simulink library "SUB_ECU_L4_MABX_HW_Interface_PIC_PB"  (R2018a)
settings: Solver=VariableStepAuto  StartTime=0.0  StopTime=10.0  RelTol=1e-3
PostLoadFcn:
  | , if any(exist('dsrtsu_mdlpostloadfcn', 'file') == [2, 3, 6]), try dsrtsu_mdlpostloadfcn('Execute', bdroot); catch fprintf('Error in PostLoadFcn (dsrtsu_mdlpostloadfcn) for model "%s":\n %s\n', bdroot, lasterr); end, end,
undefined symbols (not defined in the file or in its folder): CANR_PROPB_REAX_3_13_CHANNEL_APV, CANR_PROPB_REAX_4_13_CHANNEL_APV, CANR_PROPB_XPR_1_50_CHANNEL_APV, ENUM_CAN_RX_T, ENUM_CAN_TX_T, ENUM_REAX_OPERATION_MODE_T, ENUM_SIGNAL_HEALTH_T, ENUM_XBR_CONTROL_MODE_T, ENUM_XBR_EBI_MODE_T, ENUM_XBR_PASS_THROUGH_ACTIVE_T, ENUM_XBR_PRIORITY_T, ENUM_XPR_INHIBIT_PARK_MANUAL_T, ENUM_XPR_INHIBIT_UNPARK_MANUAL_T, ENUM_XPR_PARK_MANUAL_T, ENUM_XPR_UNPARK_MANUAL_T, PROPB_REAX_1_E4_DES_POS_SIG_SRC_APV, PROPB_REAX_1_E4_DESIRED_OPMODE_APV, PROPB_REAX_1_E4_DESIRED_POSITION_APV, PROPB_REAX_CHANNEL_APV, ptc_matlab_lib
libraries: PTC_MBDS_LIB x293, rtican x158, simulink x61, EmE_MBD_Blockset x38, rti1401lib_dio_type4 x14, simulink_need_slupdate x7, $bdroot x5, rti1401lib_adc_type4 x3, rtmapslib x3, dsa_tcpip_lib x2, SUB_ECU_L4_MABX_HW_Interface_PTC_1571 x1, rtitasklib x1
(part 32 of 49)

== system SUB_ECU_L4_MABX_HW_Interface_PIC_PB/INPUTS_PIC_PB/CAN_PIC_PB/CAN_RX_EBC1_0B/RX_CAN_1_EBC1 ==
  Enable : Inport
  Bus Creator3 : BusCreator  Inputs=25
  Data Type Conversion10 : DataTypeConversion  OutDataTypeStr=double  SaturateOnIntegerOverflow=on
  Data Type Conversion8 : DataTypeConversion  OutDataTypeStr=boolean  SaturateOnIntegerOverflow=on
  Data Type Conversion9 : DataTypeConversion  OutDataTypeStr=double  SaturateOnIntegerOverflow=on
  EBC1_0B : rtican/RTICAN Receive (RX)   Reserved1=[]  Reserved2=[]  Reserved3=[]  Reserved4=[]  SfcnMessage=[]  Msg_Struct=[]  BoardTypeNo=[]  BoardNo=[]  ChannelNo=[]  Parameters=[]  DialogFcn=[]  UnitName=[]  Revision=[]  UnitValues=[]  DSProperties=struct('RTI',struct('Version',uint32(5),'BlockType',struct('isSLSource',uint8(1),'isSLSink',uint8(1),'isHWSource',uint8(0),'isHWSink',uint8(0),'isSetup',uint8(0),'isInline',uint8(1),'isNonInline',uint8(0),'isInterrupt',uint8(0),'isChannelwise',uint8(0)),'IOBoardType','RTICAN','UnitType','MESSAGE','Identifier','RX','DialogType','MSVC','BlockSet','RTICAN','SlaveProcessor','CAN'))  RTIBlockInterface=struct('OutputPortsWidth',int32([1 1 1 1 1 1 1 1 1 1 1 1 1 1 1 1 1 1 1 1 1 1 1 1 1]),'OutputPortsActive',ones(1,25),'OutputPortsName',{{'ASREngCtrlActive','ASRBrakeCtrlActive','AntiLockBrakingActive','EBSBrakeSwitch','BrakePedalPos','ABSOffroadSwitch','ASROffroadSwitch','ASRHillHolderSwitch','TractionCtrlOverrideSwitch','AccelInterlockSwitch','EngDerateSwitch','EngAuxShutdownSwitch','RemoteAccelEnableSwitch','EngRetarderSelection','ABSFullyOperational','EBSRedWarningSignal','ABS_EBSAmberWarningSignal','ATC_ASRInformationSignal','SrcAddrssOfCtrllngDvcFrBrkCntrl','HaltBrakeSwitch','TrailerABSStatus','TrctrMntdTrilerABSWarningSignal',['RX status'],['RX time'],['RX delta time']}},'OutputPortsDataType',{{'SS_DOUBLE','SS_DOUBLE','SS_DOUBLE','SS_DOUBLE','SS_DOUBLE','SS_DOUBLE','SS_DOUBLE','SS_DOUBLE','SS_DOUBLE','SS_DOUBLE','SS_DOUBLE','SS_DOUBLE','SS_DOUBLE','SS_DOUBLE','SS_DOUBLE','SS_DOUBLE','SS_DOUBLE','SS_DOUBLE','SS_DOUBLE','SS_DOUBLE','SS_DOUBLE','SS_DOUBLE','SS_DOUBLE','SS_DOUBLE','SS_DOUBLE'}},'OutputPortsLabel',{{'ASREngCtrlActive','ASRBrakeCtrlActive','AntiLockBrakingActive','EBSBrakeSwitch','BrakePedalPos','ABSOffroadSwitch','ASROffroadSwitch','ASRHillHolderSwitch','TractionCtrlOverrideSwitch','AccelInterlockSwitch','EngDerateSwitch','EngAuxShutdownSwitch','RemoteAccelEnableSwitch','EngRetarderSelection','ABSFullyOperational','EBSRedWarningSignal','ABS_EBSAmberWarningSignal','ATC_ASRInformationSignal','SrcAddrssOfCtrllngDvcFrBrkCntrl','HaltBrakeSwitch','TrailerABSStatus','TrctrMntdTrilerABSWarningSignal','','',''}},'OutputPortsLabelMode','ON','InputPortsWidth',int32(0),'InputPortsActive',0,'DialogFcn','rtican_message_interface_gui','BlockDisplay',{{'','center'}},'IconTransparency','on','ParameterTunableNames',{{}},'InitLevel',3,'BlockName',struct('Token',{{'EBC1_0B'}}),'SampleTime',{{-1}},'TriggerPort',{{'none'}},'EnablePort',{{'yes'}})  RTIBlockParameters=struct('BoardTypeNo',{{1,'OFF',[]}},'BoardNo',{{1,'ON',[1 16]}},'ChannelNo',{{1,'ON',[1 2]}},'Parameters',{{struct('DataFileSupport',struct('DataFileSelectedMaster',1,'DataFileSelectedLocal',0,'DataFileName','c:\localdata\chris\advanced_tech\adas\level4_rcp\truck1571\dbc\mabx_can1.dbc|','DataFileDate',{{{['02-May-2017 14:24:53']},{['10-Feb-2017 15:17:28']}}},'SelectedFile',['<no file selected>']),'Options',struct('StatusSelected',1,'TimeSelected',1,'DeltaTimeSelected',1,'BytePortSelected',0,'MessageLengthSelected',0,'TriggerPort',struct('Selected',0,'TriggerType',0),'UserCoding',struct('Selected',0,'InterfaceFile','UserDecodingFile','FcnName','UserDecodeFcn','InportSelected',0,'InportWidth',1,'OutportSelected',0,'OutportWidth',1),'EnablePortSelected',1,'SignalOnPortnameSelected',1,'UseRXService',1),'Message',struct('MsgOnBlocknameSelected',1,'MsgName','EBC1_0B','MsgIdFormat',1,'MsgId',418382091,'MsgLength',8,'NumSignals',22,'SampleTime',-1,'Signal',struct('SgnName',{'ASREngCtrlActive','ASRBrakeCtrlActive','AntiLockBrakingActive','EBSBrakeSwitch','BrakePedalPos','ABSOffroadSwitch','ASROffroadSwitch','ASRHillHolderSwitch','TractionCtrlOverrideSwitch','AccelInterlockSwitch','EngDerateSwitch','EngAuxShutdownSwitch','RemoteAccelEnableSwitch','EngRetarderSelection','ABSFullyOperational','EBSRedWarningSignal','ABS_EBSAmberWarningSignal','ATC_ASRInformationSignal','SrcAddrssOfCtrllngDvcFrBrkCntrl','HaltBrakeSwitch','TrailerABSStatus','TrctrMntdTrilerABSWarningSignal'},'SgnStartBit',{0,2,4,6,8,16,18,20,22,24,26,28,30,32,40,42,44,46,48,58,60,62},'SgnLength',{2,2,2,2,8,2,2,2,2,2,2,2,2,8,2,2,2,2,8,2,2,2},'SgnType',{0,0,0,0,0,0,0,0,0,0,0,0,0,0,0,0,0,0,0,0,0,0},'ModeValue',{-1,-1,-1,-1,-1,-1,-1,-1,-1,-1,-1,-1,-1,-1,-1,-1,-1,-1,-1,-1,-1,-1},'DataType',{0,0,0,0,0,0,0,0,0,0,0,0,0,0,0,0,0,0,0,0,0,0},'ByteLayout',{0,0,0,0,0,0,0,0,0,0,0,0,0,0,0,0,0,0,0,0,0,0},'Factor',{1,1,1,1,0.4,1,1,1,1,1,1,1,1,0.4,1,1,1,1,1,1,1,1},'Offset',{0,0,0,0,0,0,0,0,0,0,0,0,0,0,0,0,0,0,0,0,0,0},'SgnComment',{{['State signal which indicates that ASR engine control has been commanded to be active.']},{['State signal which indicates that ASR brake control is active.']},{['State signal which indicates that the ABS is active.']},{['Switch signal which indicates that the brake pedal is being pressed.']},{['Ratio of brake pedal position to maximum pedal position.']},{['Switch signal which indicates the position of the ABS off-road switch.']},{['Switch signal which indicates the position of the ASR off-road switch.']},{['Switch signal which indicates the position of the ASR “hill holder” switch.']},{['Switch signal which indicates the position of the traction control override switch.']},{['Switch signal used to disable the accelerator and remote accelerator inputs, causing the engine to return to idle.']},{['Switch signal used to activate the torque limiting feature of the engine.']},{['Switch signal which requests that all engine fueling stop.']},{['Switch signal which indicates that the remote accelerator has been enabled and controls the engine.']},{['The position of the operator controlled selector, expressed as a percentage and determined by the ratio of the current']},{['Signal which indicates whether an ABS system is fully operational or whether its functionality is reduced by a defect or by']},{['This parameter commands the EBS red optical warning signal']},{['This parameter commands the ABS/EBS amber/yellow optical warning signal']},{['This parameter commands the ATC/ASR driver information signal, for example a dash lamp.']},{['The source address of the SAE J1939 device currently controlling the brake system.']},{['Switch signal which indicates the position of the halt brake switch.']},{['State signal which indicates that ABS in the trailer is actively controlling the brakes.']},{['This parameter commands the tractor-mounted trailer ABS optical warning signal.']}},'SgnUnit',{'','','','','%','','','','','','','','','%','','','','','','','',''},'Min',{0,0,0,0,0,0,0,0,0,0,0,0,0,0,0,0,0,0,0,0,0,0},'Max',{3,3,3,3,100,3,3,3,3,3,3,3,3,100,3,3,3,3,255,3,3,3},'SLDataType',{'SS_DOUBLE','SS_DOUBLE','SS_DOUBLE','SS_DOUBLE','SS_DOUBLE','SS_DOUBLE','SS_DOUBLE','SS_DOUBLE','SS_DOUBLE','SS_DOUBLE','SS_DOUBLE','SS_DOUBLE','SS_DOUBLE','SS_DOUBLE','SS_DOUBLE','SS_DOUBLE','SS_DOUBLE','SS_DOUBLE','SS_DOUBLE','SS_DOUBLE','SS_DOUBLE','SS_DOUBLE'}),'MsgIdNumFormat',1,'MsgComment',{{['Electronic Brake Controller 1']}}),'Version',1.2,'general',struct('isFromLib',0)),'OFF',[]}},'GroupId',{{struct('Group',{{'RTICAN'}},'No',1,'Behavior',{{'NAMECHANGE'}},'BlockType',{{'SINK'}},'NameChangeFlag',0),'OFF',[]}},'SFcnRTICANMessage',{{struct('MsgType','RX','SFcnPortType','Scalar','MsgName','EBC1_0B','MsgIdFormat','XTD','MsgId',418382091,'MsgLength',8,'NumSignals',22,'SampleTime',-1,'Signal',struct('SgnName',{'ASREngCtrlActive','ASRBrakeCtrlActive','AntiLockBrakingActive','EBSBrakeSwitch','BrakePedalPos','ABSOffroadSwitch','ASROffroadSwitch','ASRHillHolderSwitch','TractionCtrlOverrideSwitch','AccelInterlockSwitch','EngDerateSwitch','EngAuxShutdownSwitch','RemoteAccelEnableSwitch','EngRetarderSelection','ABSFullyOperational','EBSRedWarningSignal','ABS_EBSAmberWarningSignal','ATC_ASRInformationSignal','SrcAddrssOfCtrllngDvcFrBrkCntrl','HaltBrakeSwitch','TrailerABSStatus','TrctrMntdTrilerABSWarningSignal'},'SgnStartBit',{0,2,4,6,8,16,18,20,22,24,26,28,30,32,40,42,44,46,48,58,60,62},'SgnLength',{2,2,2,2,8,2,2,2,2,2,2,2,2,8,2,2,2,2,8,2,2,2},'SgnType',{'standard','standard','standard','standard','standard','standard','standard','standard','standard','standard','standard','standard','standard','standard','standard','standard','standard','standard','standard','standard','standard','standard'},'ModeValue',{-1,-1,-1,-1,-1,-1,-1,-1,-1,-1,-1,-1,-1,-1,-1,-1,-1,-1,-1,-1,-1,-1},'DataType',{['unsigned int'],['unsigned int'],['unsigned int'],['unsigned int'],['unsigned int'],['unsigned int'],['unsigned int'],['unsigned int'],['unsigned int'],['unsigned int'],['unsigned int'],['unsigned int'],['unsigned int'],['unsigned int'],['unsigned int'],['unsigned int'],['unsigned int'],['unsigned int'],['unsigned int'],['unsigned int'],['unsigned int'],['unsigned int']},'ByteLayout',{['little endian'],['little endian'],['little endian'],['little endian'],['little endian'],['little endian'],['little endian'],['little endian'],['little endian'],['little endian'],['little endian'],['little endian'],['little endian'],['little endian'],['little endian'],['little endian'],['little endian'],['little endian'],['little endian'],['little endian'],['little endian'],['little endian']},'Factor',{1,1,1,1,0.4,1,1,1,1,1,1,1,1,0.4,1,1,1,1,1,1,1,1},'Offset',{0,0,0,0,0,0,0,0,0,0,0,0,0,0,0,0,0,0,0,0,0,0},'SLDataType',{'SS_DOUBLE','SS_DOUBLE','SS_DOUBLE','SS_DOUBLE','SS_DOUBLE','SS_DOUBLE','SS_DOUBLE','SS_DOUBLE','SS_DOUBLE','SS_DOUBLE','SS_DOUBLE','SS_DOUBLE','SS_DOUBLE','SS_DOUBLE','SS_DOUBLE','SS_DOUBLE','SS_DOUBLE','SS_DOUBLE','SS_DOUBLE','SS_DOUBLE','SS_DOUBLE','SS_DOUBLE'}),'StatusSelected','yes','TimeSelected','yes','DeltaTimeSelected','yes','BytePortSelected','no','MessageLengthSelected','no','TriggerPort',struct('Selected','no','TriggerType',0),'UserCoding',struct('Selected','no','InterfaceFile','UserDecodingFile','FcnName','UserDecodeFcn','InportSelected','no','InportWidth',1,'OutportSelected','no','OutportWidth',1),'EnablePortSelected','yes','UseRXService','yes','BoardType','DS1','BoardNo',3,'ControllerNo',1),'OFF',[]}},'TLCFileName',{{'rtican_rx_message','OFF',[]}})  RTISFcnParameters=struct('SFcnRTICANMessage','struct','TLCFileName','char')  RTIBlockParaDefault=struct('BoardTypeNo',4302,'BoardNo',1,'ChannelNo',1,'Parameters',struct('DataFileSupport',struct('DataFileSelectedMaster',0,'DataFileSelectedLocal',0,'DataFileName','','DataFileDate','','SelectedFile',['<no file selected>']),'Options',struct('StatusSelected',1,'TimeSelected',1,'DeltaTimeSelected',1,'BytePortSelected',0,'MessageLengthSelected',0,'TriggerPort',struct('Selected',0,'TriggerType','rising'),'UserCoding',struct('Selected',0,'InterfaceFile','UserDecodingFile','FcnName','UserDecodeFcn','InportSelected',0,'InportWidth',1,'OutportSelected',0,'OutportWidth',1),'EnablePortSelected',0,'SignalOnPortnameSelected',1,'UseRXService',0),'Message',struct('MsgOnBlocknameSelected',0,'MsgName',['RX Message'],'MsgIdFormat',0,'MsgId',100,'MsgLength',8,'NumSignals',1,'SampleTime',-1,'Signal',struct('SgnName',['RX signal'],'SgnStartBit',0,'SgnLength',8,'SgnType',0,'ModeValue',-1,'DataType',0,'SLDataType','SS_DOUBLE','ByteLayout',0,'Factor',1,'Offset',0,'Min',0,'Max',255,'SgnComment',{{}},'SgnUnit',''),'MsgIdNumFormat',0,'MsgComment',{{''}}),'Version',1.2,'general',struct('isFromLib',1)),'GroupId',struct('Group',{{'RTICAN'}},'No',1,'Behavior',{{'NAMECHANGE'}},'BlockType',{{'SINK'}},'NameChangeFlag',0),'SFcnRTICANMessage',struct('MsgType','RX','MsgName',['RX Message'],'MsgIdFormat','STD','MsgId',100,'MsgLength',8,'NumSignals',1,'SampleTime',-1,'Signal',struct('SgnName',['RX signal'],'SgnStartBit',0,'SgnLength',8,'SgnType','standard','ModeValue',-1,'DataType',['unsigned int'],'ByteLayout',['little endian'],'SLDataType','SS_DOUBLE','Factor',1,'Offset',0),'StatusSelected','yes','TimeSelected','yes','DeltaTimeSelected','yes','BytePortSelected','no','MessageLengthSelected','no','EnablePortSelected','no','UserCoding',struct('Selected','no','InterfaceFile','UserDecodingFile','FcnName','UserDecodeFcn','InportSelected','no','InportWidth',1,'OutportSelected','no','OutportWidth',1),'TriggerPort',struct('Selected','no','TriggerType','rising'),'UseRXService','no','BoardType','DS4302','BoardNo',1,'ControllerNo',1,'SFcnPortType','Scalar'),'TLCFileName','rtican_rx_message')
      settings: AttributesFormatString=Group Id: RTICAN1\n  SourceProductName=dSPACE RTI CAN Blockset
  EBC1_0B_ : Outport
  wires:
  EBC1_0B/7 -> Bus Creator3/7  "ASROffroadSwitch"
  EBC1_0B/6 -> Bus Creator3/6  "ABSOffroadSwitch"
  EBC1_0B/5 -> Bus Creator3/5  "BrakePedalPos"
  EBC1_0B/4 -> Bus Creator3/4  "EBSBrakeSwitch"
  EBC1_0B/3 -> Bus Creator3/3  "AntiLockBrakingActive"
  EBC1_0B/2 -> Bus Creator3/2  "ASRBrakeCtrlActive"
  EBC1_0B/1 -> Bus Creator3/1  "ASREngCtrlActive"
  EBC1_0B/9 -> Bus Creator3/9  "TractionCtrlOverrideSwitch"
  EBC1_0B/22 -> Bus Creator3/22  "TrctrMntdTrilerABSWarningSignal"
  EBC1_0B/21 -> Bus Creator3/21  "TrailerABSStatus"
  EBC1_0B/20 -> Bus Creator3/20  "HaltBrakeSwitch"
  EBC1_0B/19 -> Bus Creator3/19  "SrcAddrssOfCtrllngDvcFrBrkCntrl"
  EBC1_0B/18 -> Bus Creator3/18  "ATC_ASRInformationSignal"
  EBC1_0B/17 -> Bus Creator3/17  "ABS_EBSAmberWarningSignal"
  EBC1_0B/16 -> Bus Creator3/16  "EBSRedWarningSignal"
  EBC1_0B/15 -> Bus Creator3/15  "ABSFullyOperational"
  EBC1_0B/14 -> Bus Creator3/14  "EngRetarderSelection"
  EBC1_0B/13 -> Bus Creator3/13  "RemoteAccelEnableSwitch"
  EBC1_0B/12 -> Bus Creator3/12  "EngAuxShutdownSwitch"
  EBC1_0B/11 -> Bus Creator3/11  "EngDerateSwitch"
  EBC1_0B/10 -> Bus Creator3/10  "AccelInterlockSwitch"
  EBC1_0B/8 -> Bus Creator3/8  "ASRHillHolderSwitch"
  Data Type Conversion9/1 -> Bus Creator3/24  "RX_time"
  Data Type Conversion10/1 -> Bus Creator3/25  "RX_delta_time"
  Data Type Conversion8/1 -> Bus Creator3/23  "RX_status"
  EBC1_0B/23 -> Data Type Conversion8/1
  EBC1_0B/24 -> Data Type Conversion9/1
  EBC1_0B/25 -> Data Type Conversion10/1
  Enable/1 -> EBC1_0B/Enable
  Bus Creator3/1 -> EBC1_0B_/1  "EBC1_0B"

== system SUB_ECU_L4_MABX_HW_Interface_PIC_PB/INPUTS_PIC_PB/CAN_PIC_PB/CAN_RX_EBC1_8B/RX_CAN_5_EBC1 ==
  Enable : Inport
  Bus Creator3 : BusCreator  Inputs=25
  Data Type Conversion10 : DataTypeConversion  OutDataTypeStr=double  SaturateOnIntegerOverflow=on
  Data Type Conversion8 : DataTypeConversion  OutDataTypeStr=boolean  SaturateOnIntegerOverflow=on
  Data Type Conversion9 : DataTypeConversion  OutDataTypeStr=double  SaturateOnIntegerOverflow=on
  EBC1_0B : rtican/RTICAN Receive (RX)   Reserved1=[]  Reserved2=[]  Reserved3=[]  Reserved4=[]  SfcnMessage=[]  Msg_Struct=[]  BoardTypeNo=[]  BoardNo=[]  ChannelNo=[]  Parameters=[]  DialogFcn=[]  UnitName=[]  Revision=[]  UnitValues=[]  DSProperties=struct('RTI',struct('Version',uint32(5),'BlockType',struct('isSLSource',uint8(1),'isSLSink',uint8(1),'isHWSource',uint8(0),'isHWSink',uint8(0),'isSetup',uint8(0),'isInline',uint8(1),'isNonInline',uint8(0),'isInterrupt',uint8(0),'isChannelwise',uint8(0)),'IOBoardType','RTICAN','UnitType','MESSAGE','Identifier','RX','DialogType','MSVC','BlockSet','RTICAN','SlaveProcessor','CAN'))  RTIBlockInterface=struct('OutputPortsWidth',int32([1 1 1 1 1 1 1 1 1 1 1 1 1 1 1 1 1 1 1 1 1 1 1 1 1]),'OutputPortsActive',ones(1,25),'OutputPortsName',{{'ASREngCtrlActive','ASRBrakeCtrlActive','AntiLockBrakingActive','EBSBrakeSwitch','BrakePedalPos','ABSOffroadSwitch','ASROffroadSwitch','ASRHillHolderSwitch','TractionCtrlOverrideSwitch','AccelInterlockSwitch','EngDerateSwitch','EngAuxShutdownSwitch','RemoteAccelEnableSwitch','EngRetarderSelection','ABSFullyOperational','EBSRedWarningSignal','ABS_EBSAmberWarningSignal','ATC_ASRInformationSignal','SrcAddrssOfCtrllngDvcFrBrkCntrl','HaltBrakeSwitch','TrailerABSStatus','TrctrMntdTrilerABSWarningSignal',['RX status'],['RX time'],['RX delta time']}},'OutputPortsDataType',{{'SS_DOUBLE','SS_DOUBLE','SS_DOUBLE','SS_DOUBLE','SS_DOUBLE','SS_DOUBLE','SS_DOUBLE','SS_DOUBLE','SS_DOUBLE','SS_DOUBLE','SS_DOUBLE','SS_DOUBLE','SS_DOUBLE','SS_DOUBLE','SS_DOUBLE','SS_DOUBLE','SS_DOUBLE','SS_DOUBLE','SS_DOUBLE','SS_DOUBLE','SS_DOUBLE','SS_DOUBLE','SS_DOUBLE','SS_DOUBLE','SS_DOUBLE'}},'OutputPortsLabel',{{'ASREngCtrlActive','ASRBrakeCtrlActive','AntiLockBrakingActive','EBSBrakeSwitch','BrakePedalPos','ABSOffroadSwitch','ASROffroadSwitch','ASRHillHolderSwitch','TractionCtrlOverrideSwitch','AccelInterlockSwitch','EngDerateSwitch','EngAuxShutdownSwitch','RemoteAccelEnableSwitch','EngRetarderSelection','ABSFullyOperational','EBSRedWarningSignal','ABS_EBSAmberWarningSignal','ATC_ASRInformationSignal','SrcAddrssOfCtrllngDvcFrBrkCntrl','HaltBrakeSwitch','TrailerABSStatus','TrctrMntdTrilerABSWarningSignal','','',''}},'OutputPortsLabelMode','ON','InputPortsWidth',int32(0),'InputPortsActive',0,'DialogFcn','rtican_message_interface_gui','BlockDisplay',{{'','center'}},'IconTransparency','on','ParameterTunableNames',{{}},'InitLevel',3,'BlockName',struct('Token',{{'EBC1_0B'}}),'SampleTime',{{-1}},'TriggerPort',{{'none'}},'EnablePort',{{'yes'}})  RTIBlockParameters=struct('BoardTypeNo',{{1,'OFF',[]}},'BoardNo',{{1,'ON',[1 16]}},'ChannelNo',{{2,'ON',[1 2]}},'Parameters',{{struct('DataFileSupport',struct('DataFileSelectedMaster',1,'DataFileSelectedLocal',0,'DataFileName',['c:\users\gavin.coelho\repos\l4 svn\branches\gennaro\project_l4\src\projectlibrary\dbc\mabx_can2.dbc|'],'DataFileDate',{{{['02-May-2017 14:24:53']},{['10-Feb-2017 15:17:28']}}},'SelectedFile',['<no file selected>']),'Options',struct('StatusSelected',1,'TimeSelected',1,'DeltaTimeSelected',1,'BytePortSelected',0,'MessageLengthSelected',0,'TriggerPort',struct('Selected',0,'TriggerType',0),'UserCoding',struct('Selected',0,'InterfaceFile','UserDecodingFile','FcnName','UserDecodeFcn','InportSelected',0,'InportWidth',1,'OutportSelected',0,'OutportWidth',1),'EnablePortSelected',1,'SignalOnPortnameSelected',1,'UseRXService',1),'Message',struct('MsgOnBlocknameSelected',1,'MsgName','EBC1_0B','MsgIdFormat',1,'MsgId',418382219,'MsgLength',8,'NumSignals',22,'SampleTime',-1,'Signal',struct('SgnName',{'ASREngCtrlActive','ASRBrakeCtrlActive','AntiLockBrakingActive','EBSBrakeSwitch','BrakePedalPos','ABSOffroadSwitch','ASROffroadSwitch','ASRHillHolderSwitch','TractionCtrlOverrideSwitch','AccelInterlockSwitch','EngDerateSwitch','EngAuxShutdownSwitch','RemoteAccelEnableSwitch','EngRetarderSelection','ABSFullyOperational','EBSRedWarningSignal','ABS_EBSAmberWarningSignal','ATC_ASRInformationSignal','SrcAddrssOfCtrllngDvcFrBrkCntrl','HaltBrakeSwitch','TrailerABSStatus','TrctrMntdTrilerABSWarningSignal'},'SgnStartBit',{0,2,4,6,8,16,18,20,22,24,26,28,30,32,40,42,44,46,48,58,60,62},'SgnLength',{2,2,2,2,8,2,2,2,2,2,2,2,2,8,2,2,2,2,8,2,2,2},'SgnType',{0,0,0,0,0,0,0,0,0,0,0,0,0,0,0,0,0,0,0,0,0,0},'ModeValue',{-1,-1,-1,-1,-1,-1,-1,-1,-1,-1,-1,-1,-1,-1,-1,-1,-1,-1,-1,-1,-1,-1},'DataType',{0,0,0,0,0,0,0,0,0,0,0,0,0,0,0,0,0,0,0,0,0,0},'ByteLayout',{0,0,0,0,0,0,0,0,0,0,0,0,0,0,0,0,0,0,0,0,0,0},'Factor',{1,1,1,1,0.4,1,1,1,1,1,1,1,1,0.4,1,1,1,1,1,1,1,1},'Offset',{0,0,0,0,0,0,0,0,0,0,0,0,0,0,0,0,0,0,0,0,0,0},'SgnComment',{{['State signal which indicates that ASR engine control has been commanded to be active.']},{['State signal which indicates that ASR brake control is active.']},{['State signal which indicates that the ABS is active.']},{['Switch signal which indicates that the brake pedal is being pressed.']},{['Ratio of brake pedal position to maximum pedal position.']},{['Switch signal which indicates the position of the ABS off-road switch.']},{['Switch signal which indicates the position of the ASR off-road switch.']},{['Switch signal which indicates the position of the ASR “hill holder” switch.']},{['Switch signal which indicates the position of the traction control override switch.']},{['Switch signal used to disable the accelerator and remote accelerator inputs, causing the engine to return to idle.']},{['Switch signal used to activate the torque limiting feature of the engine.']},{['Switch signal which requests that all engine fueling stop.']},{['Switch signal which indicates that the remote accelerator has been enabled and controls the engine.']},{['The position of the operator controlled selector, expressed as a percentage and determined by the ratio of the current']},{['Signal which indicates whether an ABS system is fully operational or whether its functionality is reduced by a defect or by']},{['This parameter commands the EBS red optical warning signal']},{['This parameter commands the ABS/EBS amber/yellow optical warning signal']},{['This parameter commands the ATC/ASR driver information signal, for example a dash lamp.']},{['The source address of the SAE J1939 device currently controlling the brake system.']},{['Switch signal which indicates the position of the halt brake switch.']},{['State signal which indicates that ABS in the trailer is actively controlling the brakes.']},{['This parameter commands the tractor-mounted trailer ABS optical warning signal.']}},'SgnUnit',{'','','','','%','','','','','','','','','%','','','','','','','',''},'Min',{0,0,0,0,0,0,0,0,0,0,0,0,0,0,0,0,0,0,0,0,0,0},'Max',{3,3,3,3,100,3,3,3,3,3,3,3,3,100,3,3,3,3,255,3,3,3},'SLDataType',{'SS_DOUBLE','SS_DOUBLE','SS_DOUBLE','SS_DOUBLE','SS_DOUBLE','SS_DOUBLE','SS_DOUBLE','SS_DOUBLE','SS_DOUBLE','SS_DOUBLE','SS_DOUBLE','SS_DOUBLE','SS_DOUBLE','SS_DOUBLE','SS_DOUBLE','SS_DOUBLE','SS_DOUBLE','SS_DOUBLE','SS_DOUBLE','SS_DOUBLE','SS_DOUBLE','SS_DOUBLE'}),'MsgIdNumFormat',1,'MsgComment',{{['Electronic Brake Controller 1']}}),'Version',1.2,'general',struct('isFromLib',0)),'OFF',[]}},'GroupId',{{struct('Group',{{'RTICAN'}},'No',2,'Behavior',{{'NAMECHANGE'}},'BlockType',{{'SINK'}},'NameChangeFlag',0),'OFF',[]}},'SFcnRTICANMessage',{{struct('MsgType','RX','SFcnPortType','Scalar','MsgName','EBC1_0B','MsgIdFormat','XTD','MsgId',418382219,'MsgLength',8,'NumSignals',22,'SampleTime',-1,'Signal',struct('SgnName',{'ASREngCtrlActive','ASRBrakeCtrlActive','AntiLockBrakingActive','EBSBrakeSwitch','BrakePedalPos','ABSOffroadSwitch','ASROffroadSwitch','ASRHillHolderSwitch','TractionCtrlOverrideSwitch','AccelInterlockSwitch','EngDerateSwitch','EngAuxShutdownSwitch','RemoteAccelEnableSwitch','EngRetarderSelection','ABSFullyOperational','EBSRedWarningSignal','ABS_EBSAmberWarningSignal','ATC_ASRInformationSignal','SrcAddrssOfCtrllngDvcFrBrkCntrl','HaltBrakeSwitch','TrailerABSStatus','TrctrMntdTrilerABSWarningSignal'},'SgnStartBit',{0,2,4,6,8,16,18,20,22,24,26,28,30,32,40,42,44,46,48,58,60,62},'SgnLength',{2,2,2,2,8,2,2,2,2,2,2,2,2,8,2,2,2,2,8,2,2,2},'SgnType',{'standard','standard','standard','standard','standard','standard','standard','standard','standard','standard','standard','standard','standard','standard','standard','standard','standard','standard','standard','standard','standard','standard'},'ModeValue',{-1,-1,-1,-1,-1,-1,-1,-1,-1,-1,-1,-1,-1,-1,-1,-1,-1,-1,-1,-1,-1,-1},'DataType',{['unsigned int'],['unsigned int'],['unsigned int'],['unsigned int'],['unsigned int'],['unsigned int'],['unsigned int'],['unsigned int'],['unsigned int'],['unsigned int'],['unsigned int'],['unsigned int'],['unsigned int'],['unsigned int'],['unsigned int'],['unsigned int'],['unsigned int'],['unsigned int'],['unsigned int'],['unsigned int'],['unsigned int'],['unsigned int']},'ByteLayout',{['little endian'],['little endian'],['little endian'],['little endian'],['little endian'],['little endian'],['little endian'],['little endian'],['little endian'],['little endian'],['little endian'],['little endian'],['little endian'],['little endian'],['little endian'],['little endian'],['little endian'],['little endian'],['little endian'],['little endian'],['little endian'],['little endian']},'Factor',{1,1,1,1,0.4,1,1,1,1,1,1,1,1,0.4,1,1,1,1,1,1,1,1},'Offset',{0,0,0,0,0,0,0,0,0,0,0,0,0,0,0,0,0,0,0,0,0,0},'SLDataType',{'SS_DOUBLE','SS_DOUBLE','SS_DOUBLE','SS_DOUBLE','SS_DOUBLE','SS_DOUBLE','SS_DOUBLE','SS_DOUBLE','SS_DOUBLE','SS_DOUBLE','SS_DOUBLE','SS_DOUBLE','SS_DOUBLE','SS_DOUBLE','SS_DOUBLE','SS_DOUBLE','SS_DOUBLE','SS_DOUBLE','SS_DOUBLE','SS_DOUBLE','SS_DOUBLE','SS_DOUBLE'}),'StatusSelected','yes','TimeSelected','yes','DeltaTimeSelected','yes','BytePortSelected','no','MessageLengthSelected','no','TriggerPort',struct('Selected','no','TriggerType',0),'UserCoding',struct('Selected','no','InterfaceFile','UserDecodingFile','FcnName','UserDecodeFcn','InportSelected','no','InportWidth',1,'OutportSelected','no','OutportWidth',1),'EnablePortSelected','yes','UseRXService','yes','BoardType','DS1','BoardNo',3,'ControllerNo',1),'OFF',[]}},'TLCFileName',{{'rtican_rx_message','OFF',[]}})  RTISFcnParameters=struct('SFcnRTICANMessage','struct','TLCFileName','char')  RTIBlockParaDefault=struct('BoardTypeNo',4302,'BoardNo',1,'ChannelNo',1,'Parameters',struct('DataFileSupport',struct('DataFileSelectedMaster',0,'DataFileSelectedLocal',0,'DataFileName','','DataFileDate','','SelectedFile',['<no file selected>']),'Options',struct('StatusSelected',1,'TimeSelected',1,'DeltaTimeSelected',1,'BytePortSelected',0,'MessageLengthSelected',0,'TriggerPort',struct('Selected',0,'TriggerType','rising'),'UserCoding',struct('Selected',0,'InterfaceFile','UserDecodingFile','FcnName','UserDecodeFcn','InportSelected',0,'InportWidth',1,'OutportSelected',0,'OutportWidth',1),'EnablePortSelected',0,'SignalOnPortnameSelected',1,'UseRXService',0),'Message',struct('MsgOnBlocknameSelected',0,'MsgName',['RX Message'],'MsgIdFormat',0,'MsgId',100,'MsgLength',8,'NumSignals',1,'SampleTime',-1,'Signal',struct('SgnName',['RX signal'],'SgnStartBit',0,'SgnLength',8,'SgnType',0,'ModeValue',-1,'DataType',0,'SLDataType','SS_DOUBLE','ByteLayout',0,'Factor',1,'Offset',0,'Min',0,'Max',255,'SgnComment',{{}},'SgnUnit',''),'MsgIdNumFormat',0,'MsgComment',{{''}}),'Version',1.2,'general',struct('isFromLib',1)),'GroupId',struct('Group',{{'RTICAN'}},'No',1,'Behavior',{{'NAMECHANGE'}},'BlockType',{{'SINK'}},'NameChangeFlag',0),'SFcnRTICANMessage',struct('MsgType','RX','MsgName',['RX Message'],'MsgIdFormat','STD','MsgId',100,'MsgLength',8,'NumSignals',1,'SampleTime',-1,'Signal',struct('SgnName',['RX signal'],'SgnStartBit',0,'SgnLength',8,'SgnType','standard','ModeValue',-1,'DataType',['unsigned int'],'ByteLayout',['little endian'],'SLDataType','SS_DOUBLE','Factor',1,'Offset',0),'StatusSelected','yes','TimeSelected','yes','DeltaTimeSelected','yes','BytePortSelected','no','MessageLengthSelected','no','EnablePortSelected','no','UserCoding',struct('Selected','no','InterfaceFile','UserDecodingFile','FcnName','UserDecodeFcn','InportSelected','no','InportWidth',1,'OutportSelected','no','OutportWidth',1),'TriggerPort',struct('Selected','no','TriggerType','rising'),'UseRXService','no','BoardType','DS4302','BoardNo',1,'ControllerNo',1,'SFcnPortType','Scalar'),'TLCFileName','rtican_rx_message')
      settings: AttributesFormatString=Group Id: RTICAN2\n  SourceProductName=dSPACE RTI CAN Blockset
  EBC1_8B : Outport
  wires:
  Bus Creator3/1 -> EBC1_8B/1  "EBC1_8B"
  Enable/1 -> EBC1_0B/Enable
  EBC1_0B/25 -> Data Type Conversion10/1
  EBC1_0B/24 -> Data Type Conversion9/1
  EBC1_0B/23 -> Data Type Conversion8/1
  Data Type Conversion8/1 -> Bus Creator3/23  "RX_status"
  Data Type Conversion10/1 -> Bus Creator3/25  "RX_delta_time"
  Data Type Conversion9/1 -> Bus Creator3/24  "RX_time"
  EBC1_0B/8 -> Bus Creator3/8  "ASRHillHolderSwitch"
  EBC1_0B/10 -> Bus Creator3/10  "AccelInterlockSwitch"
  EBC1_0B/11 -> Bus Creator3/11  "EngDerateSwitch"
  EBC1_0B/12 -> Bus Creator3/12  "EngAuxShutdownSwitch"
  EBC1_0B/13 -> Bus Creator3/13  "RemoteAccelEnableSwitch"
  EBC1_0B/14 -> Bus Creator3/14  "EngRetarderSelection"
  EBC1_0B/15 -> Bus Creator3/15  "ABSFullyOperational"
  EBC1_0B/16 -> Bus Creator3/16  "EBSRedWarningSignal"
  EBC1_0B/17 -> Bus Creator3/17  "ABS_EBSAmberWarningSignal"
  EBC1_0B/18 -> Bus Creator3/18  "ATC_ASRInformationSignal"
  EBC1_0B/19 -> Bus Creator3/19  "SrcAddrssOfCtrllngDvcFrBrkCntrl"
  EBC1_0B/20 -> Bus Creator3/20  "HaltBrakeSwitch"
  EBC1_0B/21 -> Bus Creator3/21  "TrailerABSStatus"
  EBC1_0B/22 -> Bus Creator3/22  "TrctrMntdTrilerABSWarningSignal"
  EBC1_0B/9 -> Bus Creator3/9  "TractionCtrlOverrideSwitch"
  EBC1_0B/1 -> Bus Creator3/1  "ASREngCtrlActive"
  EBC1_0B/2 -> Bus Creator3/2  "ASRBrakeCtrlActive"
  EBC1_0B/3 -> Bus Creator3/3  "AntiLockBrakingActive"
  EBC1_0B/4 -> Bus Creator3/4  "EBSBrakeSwitch"
  EBC1_0B/5 -> Bus Creator3/5  "BrakePedalPos"
  EBC1_0B/6 -> Bus Creator3/6  "ABSOffroadSwitch"
  EBC1_0B/7 -> Bus Creator3/7  "ASROffroadSwitch"

== system SUB_ECU_L4_MABX_HW_Interface_PIC_PB/INPUTS_PIC_PB/CAN_PIC_PB/CAN_RX_EBC2_0B/RX_CAN_1 ==
  Enable : Inport
  Bus Creator3 : BusCreator  Inputs=10
  Data Type Conversion10 : DataTypeConversion  OutDataTypeStr=double  SaturateOnIntegerOverflow=on
  Data Type Conversion8 : DataTypeConversion  OutDataTypeStr=boolean  SaturateOnIntegerOverflow=on
  Data Type Conversion9 : DataTypeConversion  OutDataTypeStr=double  SaturateOnIntegerOverflow=on
  EBC2_0B1 : rtican/RTICAN Receive (RX)   Reserved1=[]  Reserved2=[]  Reserved3=[]  Reserved4=[]  SfcnMessage=[]  Msg_Struct=[]  BoardTypeNo=[]  BoardNo=[]  ChannelNo=[]  Parameters=[]  DialogFcn=[]  UnitName=[]  Revision=[]  UnitValues=[]  DSProperties=struct('RTI',struct('Version',uint32(5),'BlockType',struct('isSLSource',uint8(1),'isSLSink',uint8(1),'isHWSource',uint8(0),'isHWSink',uint8(0),'isSetup',uint8(0),'isInline',uint8(1),'isNonInline',uint8(0),'isInterrupt',uint8(0),'isChannelwise',uint8(0)),'IOBoardType','RTICAN','UnitType','MESSAGE','Identifier','RX','DialogType','MSVC','BlockSet','RTICAN','SlaveProcessor','CAN'))  RTIBlockInterface=struct('OutputPortsWidth',int32([1 1 1 1 1 1 1 1 1 1]),'OutputPortsActive',[1 1 1 1 1 1 1 1 1 1],'OutputPortsName',{{'FrontAxleSpeed','RelativeSpeedFrontAxleLeftWheel','RlativeSpeedFrontAxleRightWheel','RelativeSpeedRearAxle1LeftWheel','RlativeSpeedRearAxle1RightWheel','RelativeSpeedRearAxle2LeftWheel','RlativeSpeedRearAxle2RightWheel',['RX status'],['RX time'],['RX delta time']}},'OutputPortsDataType',{{'SS_DOUBLE','SS_DOUBLE','SS_DOUBLE','SS_DOUBLE','SS_DOUBLE','SS_DOUBLE','SS_DOUBLE','SS_DOUBLE','SS_DOUBLE','SS_DOUBLE'}},'OutputPortsLabel',{{'FrontAxleSpeed','RelativeSpeedFrontAxleLeftWheel','RlativeSpeedFrontAxleRightWheel','RelativeSpeedRearAxle1LeftWheel','RlativeSpeedRearAxle1RightWheel','RelativeSpeedRearAxle2LeftWheel','RlativeSpeedRearAxle2RightWheel','','',''}},'OutputPortsLabelMode','ON','InputPortsWidth',int32(0),'InputPortsActive',0,'DialogFcn','rtican_message_interface_gui','BlockDisplay',{{'','center'}},'IconTransparency','on','ParameterTunableNames',{{}},'InitLevel',3,'BlockName',struct('Token',{{'EBC2_0B'}}),'SampleTime',{{-1}},'TriggerPort',{{'none'}},'EnablePort',{{'yes'}})  RTIBlockParameters=struct('BoardTypeNo',{{1,'OFF',[]}},'BoardNo',{{1,'ON',[1 16]}},'ChannelNo',{{1,'ON',[1 2]}},'Parameters',{{struct('DataFileSupport',struct('DataFileSelectedMaster',1,'DataFileSelectedLocal',1,'DataFileName','c:\localdata\chris\advanced_tech\adas\level4_rcp\truck1571\dbc\j1939_famosdbcwithfusion.dbc|','DataFileDate',{{{['03-Apr-2017 12:55:40']}}},'SelectedFile','dbc\j1939_famosdbcwithfusion.dbc'),'Options',struct('StatusSelected',1,'TimeSelected',1,'DeltaTimeSelected',1,'BytePortSelected',0,'MessageLengthSelected',0,'TriggerPort',struct('Selected',0,'TriggerType',0),'UserCoding',struct('Selected',0,'InterfaceFile','UserDecodingFile','FcnName','UserDecodeFcn','InportSelected',0,'InportWidth',1,'OutportSelected',0,'OutportWidth',1),'EnablePortSelected',1,'SignalOnPortnameSelected',1,'UseRXService',1),'Message',struct('MsgOnBlocknameSelected',1,'MsgName','EBC2_0B','MsgIdFormat',1,'MsgId',419348235,'MsgLength',8,'NumSignals',7,'SampleTime',-1,'Signal',struct('SgnName',{'FrontAxleSpeed','RelativeSpeedFrontAxleLeftWheel','RlativeSpeedFrontAxleRightWheel','RelativeSpeedRearAxle1LeftWheel','RlativeSpeedRearAxle1RightWheel','RelativeSpeedRearAxle2LeftWheel','RlativeSpeedRearAxle2RightWheel'},'SgnStartBit',{0,16,24,32,40,48,56},'SgnLength',{16,8,8,8,8,8,8},'SgnType',{0,0,0,0,0,0,0},'ModeValue',{-1,-1,-1,-1,-1,-1,-1},'DataType',{0,0,0,0,0,0,0},'ByteLayout',{0,0,0,0,0,0,0},'Factor',{2^-8,2^-4,2^-4,2^-4,2^-4,2^-4,2^-4},'Offset',{0,-7.8125,-7.8125,-7.8125,-7.8125,-7.8125,-7.8125},'SgnComment',{{['The average speed of the two front wheels.']},{['The speed of the front axle, left wheel relative to the front axle speed, SPN 904.']},{['The speed of the front axle, right wheel relative to the front axle speed, SPN 904.']},{['The speed of the rear axle #1, left wheel relative to the front axle speed, SPN 904.']},{['The speed of the rear axle #1, right wheel relative to the front axle speed, SPN 904.']},{['The speed of the rear axle #2, left wheel relative to the front axle speed, SPN 904.']},{['The speed of the rear axle #2, right wheel relative to the front axle speed, SPN 904.']}},'SgnUnit',{'km/h','km/h','km/h','km/h','km/h','km/h','km/h'},'Min',{0,-7.8125,-7.8125,-7.8125,-7.8125,-7.8125,-7.8125},'Max',{250.996,7.8125,7.8125,7.8125,7.8125,7.8125,7.8125},'SLDataType',{'SS_DOUBLE','SS_DOUBLE','SS_DOUBLE','SS_DOUBLE','SS_DOUBLE','SS_DOUBLE','SS_DOUBLE'}),'MsgIdNumFormat',0,'MsgComment',{{['Wheel Speed Information']}}),'Version',1.2,'general',struct('isFromLib',0)),'OFF',[]}},'GroupId',{{struct('Group',{{'RTICAN'}},'No',1,'Behavior',{{'NAMECHANGE'}},'BlockType',{{'SINK'}},'NameChangeFlag',0),'OFF',[]}},'SFcnRTICANMessage',{{struct('MsgType','RX','SFcnPortType','Scalar','MsgName','EBC2_0B','MsgIdFormat','XTD','MsgId',419348235,'MsgLength',8,'NumSignals',7,'SampleTime',-1,'Signal',struct('SgnName',{'FrontAxleSpeed','RelativeSpeedFrontAxleLeftWheel','RlativeSpeedFrontAxleRightWheel','RelativeSpeedRearAxle1LeftWheel','RlativeSpeedRearAxle1RightWheel','RelativeSpeedRearAxle2LeftWheel','RlativeSpeedRearAxle2RightWheel'},'SgnStartBit',{0,16,24,32,40,48,56},'SgnLength',{16,8,8,8,8,8,8},'SgnType',{'standard','standard','standard','standard','standard','standard','standard'},'ModeValue',{-1,-1,-1,-1,-1,-1,-1},'DataType',{['unsigned int'],['unsigned int'],['unsigned int'],['unsigned int'],['unsigned int'],['unsigned int'],['unsigned int']},'ByteLayout',{['little endian'],['little endian'],['little endian'],['little endian'],['little endian'],['little endian'],['little endian']},'Factor',{2^-8,2^-4,2^-4,2^-4,2^-4,2^-4,2^-4},'Offset',{0,-7.8125,-7.8125,-7.8125,-7.8125,-7.8125,-7.8125},'SLDataType',{'SS_DOUBLE','SS_DOUBLE','SS_DOUBLE','SS_DOUBLE','SS_DOUBLE','SS_DOUBLE','SS_DOUBLE'}),'StatusSelected','yes','TimeSelected','yes','DeltaTimeSelected','yes','BytePortSelected','no','MessageLengthSelected','no','TriggerPort',struct('Selected','no','TriggerType',0),'UserCoding',struct('Selected','no','InterfaceFile','UserDecodingFile','FcnName','UserDecodeFcn','InportSelected','no','InportWidth',1,'OutportSelected','no','OutportWidth',1),'EnablePortSelected','yes','UseRXService','yes','BoardType','DS1','BoardNo',1,'ControllerNo',1),'OFF',[]}},'TLCFileName',{{'rtican_rx_message','OFF',[]}})  RTISFcnParameters=struct('SFcnRTICANMessage','struct','TLCFileName','char')  RTIBlockParaDefault=struct('BoardTypeNo',4302,'BoardNo',1,'ChannelNo',1,'Parameters',struct('DataFileSupport',struct('DataFileSelectedMaster',0,'DataFileSelectedLocal',0,'DataFileName','','DataFileDate','','SelectedFile',['<no file selected>']),'Options',struct('StatusSelected',1,'TimeSelected',1,'DeltaTimeSelected',1,'BytePortSelected',0,'MessageLengthSelected',0,'TriggerPort',struct('Selected',0,'TriggerType','rising'),'UserCoding',struct('Selected',0,'InterfaceFile','UserDecodingFile','FcnName','UserDecodeFcn','InportSelected',0,'InportWidth',1,'OutportSelected',0,'OutportWidth',1),'EnablePortSelected',0,'SignalOnPortnameSelected',1,'UseRXService',0),'Message',struct('MsgOnBlocknameSelected',0,'MsgName',['RX Message'],'MsgIdFormat',0,'MsgId',100,'MsgLength',8,'NumSignals',1,'SampleTime',-1,'Signal',struct('SgnName',['RX signal'],'SgnStartBit',0,'SgnLength',8,'SgnType',0,'ModeValue',-1,'DataType',0,'SLDataType','SS_DOUBLE','ByteLayout',0,'Factor',1,'Offset',0,'Min',0,'Max',255,'SgnComment',{{}},'SgnUnit',''),'MsgIdNumFormat',0,'MsgComment',{{''}}),'Version',1.2,'general',struct('isFromLib',1)),'GroupId',struct('Group',{{'RTICAN'}},'No',1,'Behavior',{{'NAMECHANGE'}},'BlockType',{{'SINK'}},'NameChangeFlag',0),'SFcnRTICANMessage',struct('MsgType','RX','MsgName',['RX Message'],'MsgIdFormat','STD','MsgId',100,'MsgLength',8,'NumSignals',1,'SampleTime',-1,'Signal',struct('SgnName',['RX signal'],'SgnStartBit',0,'SgnLength',8,'SgnType','standard','ModeValue',-1,'DataType',['unsigned int'],'ByteLayout',['little endian'],'SLDataType','SS_DOUBLE','Factor',1,'Offset',0),'StatusSelected','yes','TimeSelected','yes','DeltaTimeSelected','yes','BytePortSelected','no','MessageLengthSelected','no','EnablePortSelected','no','UserCoding',struct('Selected','no','InterfaceFile','UserDecodingFile','FcnName','UserDecodeFcn','InportSelected','no','InportWidth',1,'OutportSelected','no','OutportWidth',1),'TriggerPort',struct('Selected','no','TriggerType','rising'),'UseRXService','no','BoardType','DS4302','BoardNo',1,'ControllerNo',1,'SFcnPortType','Scalar'),'TLCFileName','rtican_rx_message')
      settings: AttributesFormatString=Group Id: RTICAN1\n  SourceProductName=dSPACE RTI CAN Blockset
  EBC2_0B : Outport
  wires:
  EBC2_0B1/7 -> Bus Creator3/7  "RlativeSpeedRearAxle2RightWheel"
  EBC2_0B1/6 -> Bus Creator3/6  "RelativeSpeedRearAxle2LeftWheel"
  EBC2_0B1/5 -> Bus Creator3/5  "RlativeSpeedRearAxle1RightWheel"
  EBC2_0B1/1 -> Bus Creator3/1  "FrontAxleSpeed"
  EBC2_0B1/3 -> Bus Creator3/3  "RlativeSpeedFrontAxleRightWheel"
  EBC2_0B1/4 -> Bus Creator3/4  "RelativeSpeedRearAxle1LeftWheel"
  EBC2_0B1/2 -> Bus Creator3/2  "RelativeSpeedFrontAxleLeftWheel"
  Data Type Conversion9/1 -> Bus Creator3/9  "RX_time"
  Data Type Conversion10/1 -> Bus Creator3/10  "RX_delta_time"
  Data Type Conversion8/1 -> Bus Creator3/8  "RX_status"
  EBC2_0B1/8 -> Data Type Conversion8/1
  EBC2_0B1/9 -> Data Type Conversion9/1
  EBC2_0B1/10 -> Data Type Conversion10/1
  Enable/1 -> EBC2_0B1/Enable
  Bus Creator3/1 -> EBC2_0B/1  "EBC2_0B"

== system SUB_ECU_L4_MABX_HW_Interface_PIC_PB/INPUTS_PIC_PB/CAN_PIC_PB/CAN_RX_EC1_00/CAN_RX_EC1_00 ==
  TPCM : Inport
  TPDT : Inport  Port=2
  timeStamp : Inport  Port=3
  Enable : EnablePort
  Bus Selector1 : BusSelector  OutputSignals=Signals.SPN2572_SequenceNumber
  Bus Selector3 : BusSelector  OutputSignals=Signals.SPN2573_PacketizedData
  Bus Selector4 : BusSelector  OutputSignals=Signals.TPCM_BAM.SPN2568_TotalNumberOfPackets
  Decode : Subsystem  TreatAsAtomicUnit=on
  Demux : Demux  Outputs=7
  Unit Delay : UnitDelay  InitialCondition=uint8(hex2dec('FF')) * ones(39, 1, 'uint8')  SampleTime=-1
  serialize_tpdt : MATLAB Function  TreatAsAtomicUnit=on
  RawData : Outport
  RX_status : Outport  Port=2
  RX_time : Outport  Port=3
  RX_delta_time : Outport  Port=4
  wires:
  timeStamp/1 -> Decode/2(timeStamp)
  Demux/3 -> serialize_tpdt/6(byte3)
  Demux/7 -> serialize_tpdt/10(byte7)
  Demux/6 -> serialize_tpdt/9(byte6)
  Demux/4 -> serialize_tpdt/7(byte4)
  Demux/5 -> serialize_tpdt/8(byte5)
  Demux/2 -> serialize_tpdt/5(byte2)
  Demux/1 -> serialize_tpdt/4(byte1)
  Bus Selector3/1 -> Demux/1  "<SPN2573_PacketizedData>"
  Decode/1(RawData) -> RawData/1  "RawData"
  Decode/3(RX_delta_time) -> RX_delta_time/1  "RX_delta_time"
  Decode/2(RX_time) -> RX_time/1  "RX_time"
  serialize_tpdt/1(RX_status) -> Decode/Enable, RX_status/1  "RX_status"
  serialize_tpdt/2(Data) -> Decode/1(Inport), Unit Delay/1
  Unit Delay/1 -> serialize_tpdt/1(data_packet_previous)
  Bus Selector4/1 -> serialize_tpdt/2(TotalNumberOfPackets)  "<SPN2568_TotalNumberOfPackets>"
  Bus Selector1/1 -> serialize_tpdt/3(SequenceNumber)  "<SPN2572_SequenceNumber>"
  [TPDT] -> Bus Selector3/1, Bus Selector1/1
  [TPCM] -> Bus Selector4/1
  TPDT/1 -> [TPDT]
  TPCM/1 -> [TPCM]
